simulink model "ss_project_observer"  (R2014b)
settings: Solver=ode45  StartTime=0.0  StopTime=10.0  RelTol=1e-3
values from neighbouring files (symbols this model uses):
  A = diag([1 1 1],1)    [list3.m]
  B = [0 0 1]'    [list3.m]
  C = [1 1 0]    [list3.m]
  F = [F1 F2 F3]    [p3ss.m]    (also in ss_observer_ref_following.m = double(nF); ss_ref_following.m = double(F))
  G = tf(1,[1 a])*tf(1,[1 b])    [freq_control.m]    (also in freqcontrol.m = tf(10,[1 0 0])*tf([1 .5],[1 2])*tf(1,[1 10]); list3.m = C*(s*I - A)^(-1)*B; p2freq.m; p3ss.m = tf([1],[1 6 11 6]))
  L = double(nL)    [ss_observer_ref_following.m]
  N = x(end)    [p3ss.m]    (also in ss_observer_ref_following.m = double(x(end)); ss_ref_following.m = double(x(end)))
settings Model: Creator=rafael  LastModifiedBy=rafael

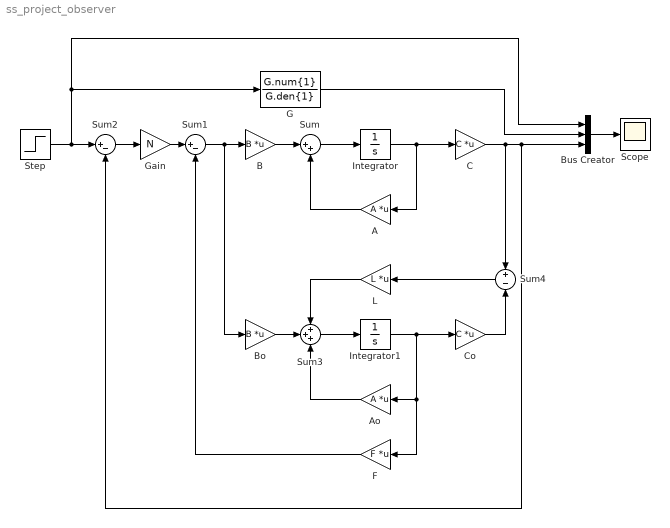
== system ss_project_observer ==
  A : Gain  Gain=A  Multiplication=Matrix(K*u) (u vector)
  Ao : Gain  Gain=A  Multiplication=Matrix(K*u) (u vector)
  B : Gain  Gain=B  Multiplication=Matrix(K*u) (u vector)
  Bo : Gain  Gain=B  Multiplication=Matrix(K*u) (u vector)
  Bus Creator : BusCreator  Inputs=3
  C : Gain  Gain=C  Multiplication=Matrix(K*u) (u vector)
  Co : Gain  Gain=C  Multiplication=Matrix(K*u) (u vector)
  F : Gain  Gain=F  Multiplication=Matrix(K*u) (u vector)
  G : TransferFcn  Numerator=G.num{1}  Denominator=G.den{1}
  Gain : Gain  Gain=N
  Integrator : Integrator
  Integrator1 : Integrator
  L : Gain  Gain=L  Multiplication=Matrix(K*u) (u vector)
  Scope : Scope
  Step : Step  SampleTime=0
  Sum : Sum  Inputs=|++
  Sum1 : Sum  Inputs=|+-
  Sum2 : Sum  Inputs=|+-
  Sum3 : Sum  Inputs=+++
  Sum4 : Sum  Inputs=+|-
  wires:
  B/1 -> Sum/1
  A/1 -> Sum/2
  Sum/1 -> Integrator/1
  Integrator/1 -> C/1, A/1
  C/1 -> Bus Creator/3, Sum2/2, Sum4/1
  Bus Creator/1 -> Scope/1
  G/1 -> Bus Creator/2
  Sum2/1 -> Gain/1
  Gain/1 -> Sum1/1
  Step/1 -> Sum2/1, Bus Creator/1, G/1
  Sum3/1 -> Integrator1/1
  Integrator1/1 -> Co/1, F/1, Ao/1
  Sum1/1 -> Bo/1, B/1
  F/1 -> Sum1/2
  Sum4/1 -> L/1
  L/1 -> Sum3/1
  Bo/1 -> Sum3/2
  Ao/1 -> Sum3/3
  Co/1 -> Sum4/2
